simulink model "ntw4_3_2"  (R2018b)
settings: Solver=VariableStepAuto  StartTime=0.0  StopTime=10.0  RelTol=1e-3
settings Model: Creator=fyna  LastModifiedBy=fyna

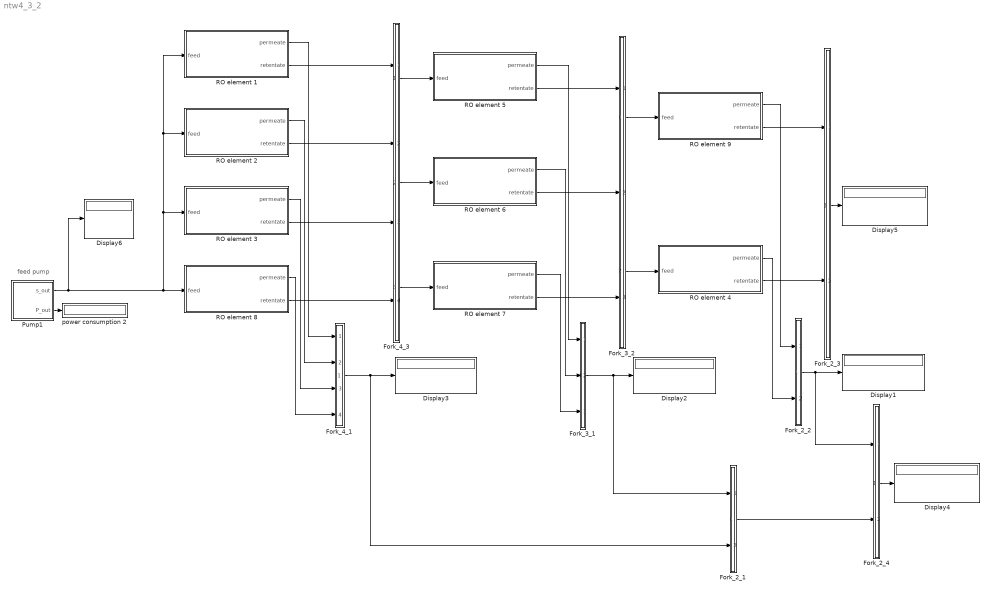
== system ntw4_3_2 ==
  note: feed pump
  Display{1..6} (6 alike) : Display
  Fork_2_1 : MATLAB Function  TreatAsAtomicUnit=on
  Fork_2_2 : MATLAB Function  TreatAsAtomicUnit=on
  Fork_2_3 : MATLAB Function  TreatAsAtomicUnit=on
  Fork_2_4 : MATLAB Function  TreatAsAtomicUnit=on
  Fork_3_1 : MATLAB Function  TreatAsAtomicUnit=on
  Fork_3_2 : MATLAB Function  TreatAsAtomicUnit=on
  Fork_4_1 : MATLAB Function  TreatAsAtomicUnit=on
  "Fork_4_3 " : MATLAB Function  TreatAsAtomicUnit=on
  Pump1 : Subsystem  mask(Hydraulic pump){q=6e3, p=15.5, c=0.0856, eta=0.8}
      mask prompts: q "volume flow rate [l/h]"; p "pressure [bar]"; c "concentration [mol/l]"; eta "efficiency"
      mask help: The hydraulic pump gerenates the hydrodynamic QPC state, through its embedded preferences. The power consumption is calculated as P = 3.6e-2*q*p/eta, [P] = kW.
      mask TypeOptions q: flow rate [l\h]/Value
      mask TypeOptions p: pressure [Pa]/Value
      mask TypeOptions c: concentration [mol//l]/Value
      mask TypeOptions eta: efficiency/Value
      mask Display: image("pumpSymbol2.png")
  RO element 1 : Subsystem  mask(8040 RO module){waterPerm=5, Value=0.995}
      mask prompts: waterPerm "water permeation coeff [lmh bar]]"; Value "salt rejection"
      mask help:
      | Reverse Osmosis module model. The permeate out-flow and feed out-flow are calculated from their respective in-flows and the membrane characteristics. A 28mil spacer is used in this module type.
      |
      | Input constants: membrane water permeability, salt rejection.
      mask TypeOptions waterPerm: waterPerm/Value
      mask TypeOptions Value: rejectionRate/Value
      mask Display: image('roSymbol.png');
  RO element 2 : Subsystem  mask(8040 RO module){waterPerm=5, Value=0.995}
      mask prompts: waterPerm "water permeation coeff [lmh bar]]"; Value "salt rejection"
      mask help:
      | Reverse Osmosis module model. The permeate out-flow and feed out-flow are calculated from their respective in-flows and the membrane characteristics. A 28mil spacer is used in this module type.
      |
      | Input constants: membrane water permeability, salt rejection.
      mask TypeOptions waterPerm: waterPerm/Value
      mask TypeOptions Value: rejectionRate/Value
      mask Display: image('roSymbol.png');
  RO element 3 : Subsystem  mask(8040 RO module){waterPerm=5, Value=0.995}
      mask prompts: waterPerm "water permeation coeff [lmh bar]]"; Value "salt rejection"
      mask help:
      | Reverse Osmosis module model. The permeate out-flow and feed out-flow are calculated from their respective in-flows and the membrane characteristics. A 28mil spacer is used in this module type.
      |
      | Input constants: membrane water permeability, salt rejection.
      mask TypeOptions waterPerm: waterPerm/Value
      mask TypeOptions Value: rejectionRate/Value
      mask Display: image('roSymbol.png');
  RO element 4 : Subsystem  mask(8040 RO module){waterPerm=5, Value=0.995}
      mask prompts: waterPerm "water permeation coeff [lmh bar]]"; Value "salt rejection"
      mask help:
      | Reverse Osmosis module model. The permeate out-flow and feed out-flow are calculated from their respective in-flows and the membrane characteristics. A 28mil spacer is used in this module type.
      |
      | Input constants: membrane water permeability, salt rejection.
      mask TypeOptions waterPerm: waterPerm/Value
      mask TypeOptions Value: rejectionRate/Value
      mask Display: image('roSymbol.png');
  RO element 5 : Subsystem  mask(8040 RO module){waterPerm=5, Value=0.995}
      mask prompts: waterPerm "water permeation coeff [lmh bar]]"; Value "salt rejection"
      mask help:
      | Reverse Osmosis module model. The permeate out-flow and feed out-flow are calculated from their respective in-flows and the membrane characteristics. A 28mil spacer is used in this module type.
      |
      | Input constants: membrane water permeability, salt rejection.
      mask TypeOptions waterPerm: waterPerm/Value
      mask TypeOptions Value: rejectionRate/Value
      mask Display: image('roSymbol.png');
  RO element 6 : Subsystem  mask(8040 RO module){waterPerm=5, Value=0.995}
      mask prompts: waterPerm "water permeation coeff [lmh bar]]"; Value "salt rejection"
      mask help:
      | Reverse Osmosis module model. The permeate out-flow and feed out-flow are calculated from their respective in-flows and the membrane characteristics. A 28mil spacer is used in this module type.
      |
      | Input constants: membrane water permeability, salt rejection.
      mask TypeOptions waterPerm: waterPerm/Value
      mask TypeOptions Value: rejectionRate/Value
      mask Display: image('roSymbol.png');
  RO element 7 : Subsystem  mask(8040 RO module){waterPerm=5, Value=0.995}
      mask prompts: waterPerm "water permeation coeff [lmh bar]]"; Value "salt rejection"
      mask help:
      | Reverse Osmosis module model. The permeate out-flow and feed out-flow are calculated from their respective in-flows and the membrane characteristics. A 28mil spacer is used in this module type.
      |
      | Input constants: membrane water permeability, salt rejection.
      mask TypeOptions waterPerm: waterPerm/Value
      mask TypeOptions Value: rejectionRate/Value
      mask Display: image('roSymbol.png');
  RO element 8 : Subsystem  mask(8040 RO module){waterPerm=5, Value=0.995}
      mask prompts: waterPerm "water permeation coeff [lmh bar]]"; Value "salt rejection"
      mask help:
      | Reverse Osmosis module model. The permeate out-flow and feed out-flow are calculated from their respective in-flows and the membrane characteristics. A 28mil spacer is used in this module type.
      |
      | Input constants: membrane water permeability, salt rejection.
      mask TypeOptions waterPerm: waterPerm/Value
      mask TypeOptions Value: rejectionRate/Value
      mask Display: image('roSymbol.png');
  RO element 9 : Subsystem  mask(8040 RO module){waterPerm=5, Value=0.995}
      mask prompts: waterPerm "water permeation coeff [lmh bar]]"; Value "salt rejection"
      mask help:
      | Reverse Osmosis module model. The permeate out-flow and feed out-flow are calculated from their respective in-flows and the membrane characteristics. A 28mil spacer is used in this module type.
      |
      | Input constants: membrane water permeability, salt rejection.
      mask TypeOptions waterPerm: waterPerm/Value
      mask TypeOptions Value: rejectionRate/Value
      mask Display: image('roSymbol.png');
  power consumption 2 : Display
  wires:
  RO element 8/2(retentate) -> "Fork_4_3 "/4(si_4)
  RO element 5/1(permeate) -> Fork_3_1/1(si_1)
  RO element 3/1(permeate) -> Fork_4_1/3(si_3)
  RO element 1/1(permeate) -> Fork_4_1/1(si_1)
  RO element 8/1(permeate) -> Fork_4_1/4(si_4)
  RO element 2/2(retentate) -> "Fork_4_3 "/2(si_2)
  Fork_4_1/1(so_1) -> Display3/1, Fork_2_1/2(si_2)
  Pump1/2(P_out) -> power consumption 2/1
  RO element 3/2(retentate) -> "Fork_4_3 "/3(si_3)
  Pump1/1(s_out) -> RO element 8/1(feed), RO element 3/1(feed), RO element 1/1(feed), RO element 2/1(feed), Display6/1
  RO element 1/2(retentate) -> "Fork_4_3 "/1(si_1)
  RO element 6/1(permeate) -> Fork_3_1/2(si_2)
  RO element 2/1(permeate) -> Fork_4_1/2(si_2)
  "Fork_4_3 "/1(so_1) -> RO element 5/1(feed)
  "Fork_4_3 "/2(so_2) -> RO element 6/1(feed)
  "Fork_4_3 "/3(so_3) -> RO element 7/1(feed)
  RO element 7/1(permeate) -> Fork_3_1/3(si_3)
  RO element 7/2(retentate) -> Fork_3_2/3(si_3)
  RO element 6/2(retentate) -> Fork_3_2/2(si_2)
  RO element 5/2(retentate) -> Fork_3_2/1(si_1)
  Fork_3_2/2(so_2) -> RO element 4/1(feed)
  Fork_3_2/1(so_1) -> RO element 9/1(feed)
  Fork_3_1/1(so_1) -> Display2/1, Fork_2_1/1(si_1)
  RO element 9/1(permeate) -> Fork_2_2/1(si_1)
  RO element 4/1(permeate) -> Fork_2_2/2(si_2)
  Fork_2_1/1(so_1) -> Fork_2_4/2(si_2)
  Fork_2_2/1(so_1) -> Display1/1, Fork_2_4/1(si_1)
  Fork_2_4/1(so_1) -> Display4/1
  RO element 9/2(retentate) -> Fork_2_3/1(si_1)
  RO element 4/2(retentate) -> Fork_2_3/2(si_2)
  Fork_2_3/1(so_1) -> Display5/1

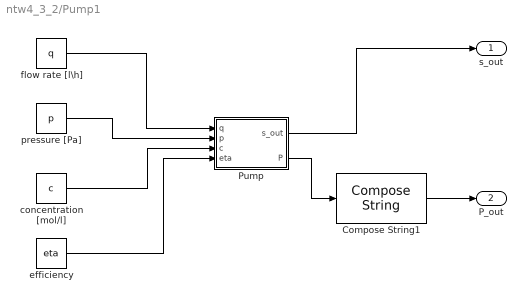
== system ntw4_3_2/Pump1 ==
  Compose String1 : ComposeString  Format='P = %.3f kW'
  Pump : MATLAB Function  TreatAsAtomicUnit=on
  concentration [mol/l] : Constant  Value=c
  efficiency : Constant  Value=eta
  flow rate [l\h] : Constant  Value=q
  pressure [Pa] : Constant  Value=p
  s_out : Outport
  P_out : Outport  Port=2
  wires:
  concentration [mol/l]/1 -> Pump/3(c)
  flow rate [l\h]/1 -> Pump/1(q)
  Pump/1(s_out) -> s_out/1
  pressure [Pa]/1 -> Pump/2(p)
  efficiency/1 -> Pump/4(eta)
  Compose String1/1 -> P_out/1
  Pump/2(P) -> Compose String1/1

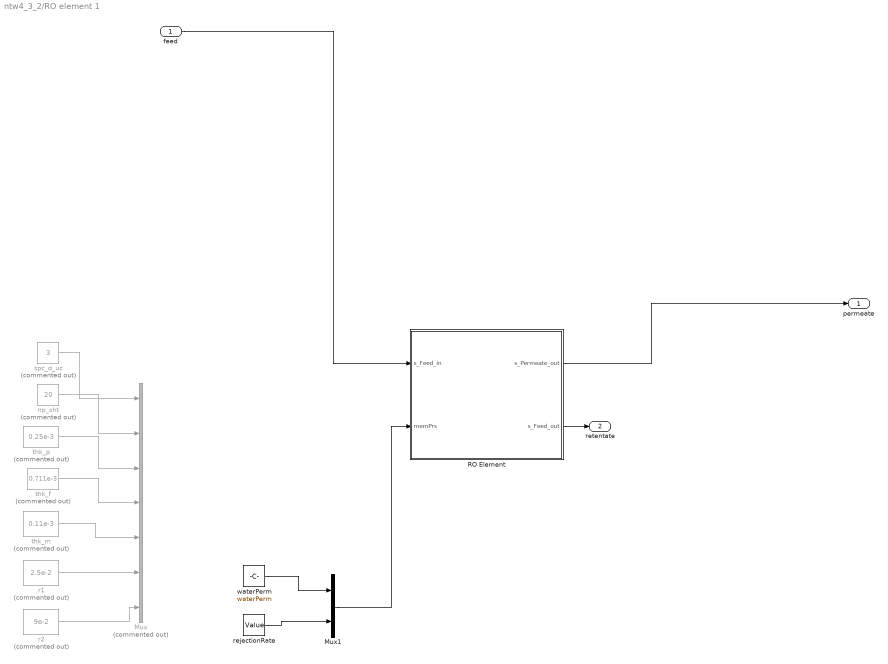
== system ntw4_3_2/RO element 1 ==
  feed : Inport
  Mux : Mux  Commented=on  Inputs=7
  Mux1 : Mux  Inputs=2
  RO Element : MATLAB Function  TreatAsAtomicUnit=on
  np_sht : Constant  Commented=on  Value=20
  r1 : Constant  Commented=on  Value=2.5e-2
  r2 : Constant  Commented=on  Value=9e-2
  rejectionRate : Constant  Value=Value
  spc_d_uc : Constant  Commented=on  Value=3
  thk_f : Constant  Commented=on  Value=0.711e-3
  thk_m : Constant  Commented=on  Value=0.11e-3
  thk_p : Constant  Commented=on  Value=0.25e-3
  waterPerm : Constant  Value=waterPerm
  permeate : Outport
  retentate : Outport  Port=2
  wires:
  spc_d_uc/1 -> Mux/1
  feed/1 -> RO Element/1(s_Feed_in)
  waterPerm/1 -> Mux1/1
  r1/1 -> Mux/6
  thk_m/1 -> Mux/5
  Mux1/1 -> RO Element/2(memPrs)
  r2/1 -> Mux/7
  RO Element/2(s_Feed_out) -> retentate/1
  rejectionRate/1 -> Mux1/2
  RO Element/1(s_Permeate_out) -> permeate/1
  thk_p/1 -> Mux/3
  thk_f/1 -> Mux/4
  np_sht/1 -> Mux/2

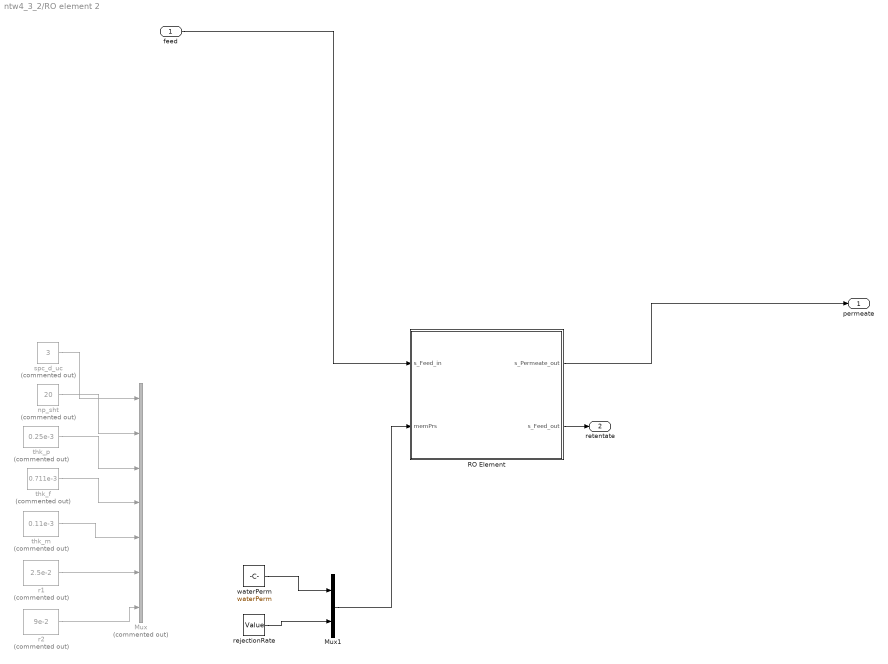
== system ntw4_3_2/RO element 2 ==
  feed : Inport
  Mux : Mux  Commented=on  Inputs=7
  Mux1 : Mux  Inputs=2
  RO Element : MATLAB Function  TreatAsAtomicUnit=on
  np_sht : Constant  Commented=on  Value=20
  r1 : Constant  Commented=on  Value=2.5e-2
  r2 : Constant  Commented=on  Value=9e-2
  rejectionRate : Constant  Value=Value
  spc_d_uc : Constant  Commented=on  Value=3
  thk_f : Constant  Commented=on  Value=0.711e-3
  thk_m : Constant  Commented=on  Value=0.11e-3
  thk_p : Constant  Commented=on  Value=0.25e-3
  waterPerm : Constant  Value=waterPerm
  permeate : Outport
  retentate : Outport  Port=2
  wires:
  spc_d_uc/1 -> Mux/1
  feed/1 -> RO Element/1(s_Feed_in)
  waterPerm/1 -> Mux1/1
  r1/1 -> Mux/6
  thk_m/1 -> Mux/5
  Mux1/1 -> RO Element/2(memPrs)
  r2/1 -> Mux/7
  RO Element/2(s_Feed_out) -> retentate/1
  rejectionRate/1 -> Mux1/2
  RO Element/1(s_Permeate_out) -> permeate/1
  thk_p/1 -> Mux/3
  thk_f/1 -> Mux/4
  np_sht/1 -> Mux/2

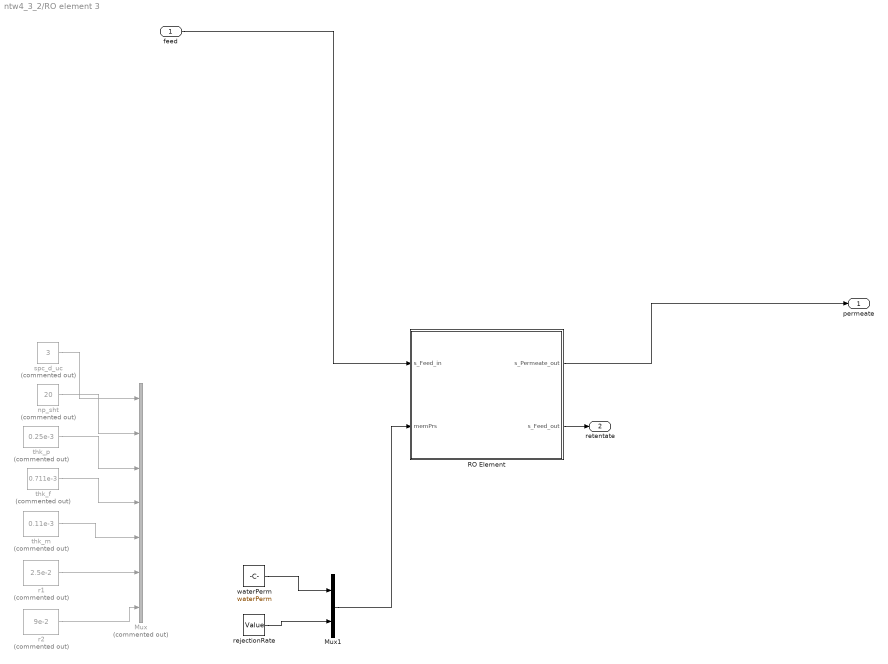
== system ntw4_3_2/RO element 3 ==
  feed : Inport
  Mux : Mux  Commented=on  Inputs=7
  Mux1 : Mux  Inputs=2
  RO Element : MATLAB Function  TreatAsAtomicUnit=on
  np_sht : Constant  Commented=on  Value=20
  r1 : Constant  Commented=on  Value=2.5e-2
  r2 : Constant  Commented=on  Value=9e-2
  rejectionRate : Constant  Value=Value
  spc_d_uc : Constant  Commented=on  Value=3
  thk_f : Constant  Commented=on  Value=0.711e-3
  thk_m : Constant  Commented=on  Value=0.11e-3
  thk_p : Constant  Commented=on  Value=0.25e-3
  waterPerm : Constant  Value=waterPerm
  permeate : Outport
  retentate : Outport  Port=2
  wires:
  spc_d_uc/1 -> Mux/1
  feed/1 -> RO Element/1(s_Feed_in)
  waterPerm/1 -> Mux1/1
  r1/1 -> Mux/6
  thk_m/1 -> Mux/5
  Mux1/1 -> RO Element/2(memPrs)
  r2/1 -> Mux/7
  RO Element/2(s_Feed_out) -> retentate/1
  rejectionRate/1 -> Mux1/2
  RO Element/1(s_Permeate_out) -> permeate/1
  thk_p/1 -> Mux/3
  thk_f/1 -> Mux/4
  np_sht/1 -> Mux/2

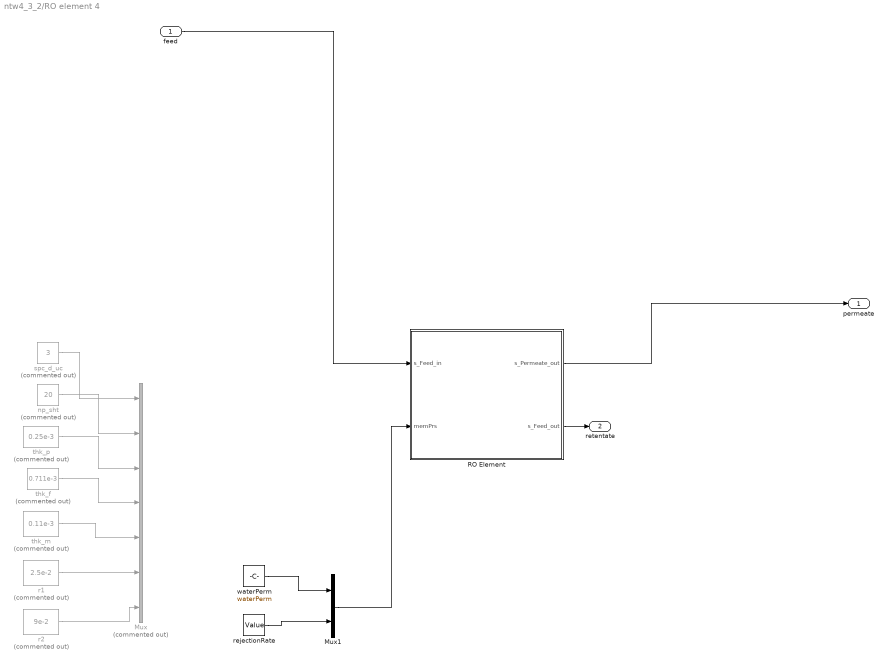
== system ntw4_3_2/RO element 4 ==
  feed : Inport
  Mux : Mux  Commented=on  Inputs=7
  Mux1 : Mux  Inputs=2
  RO Element : MATLAB Function  TreatAsAtomicUnit=on
  np_sht : Constant  Commented=on  Value=20
  r1 : Constant  Commented=on  Value=2.5e-2
  r2 : Constant  Commented=on  Value=9e-2
  rejectionRate : Constant  Value=Value
  spc_d_uc : Constant  Commented=on  Value=3
  thk_f : Constant  Commented=on  Value=0.711e-3
  thk_m : Constant  Commented=on  Value=0.11e-3
  thk_p : Constant  Commented=on  Value=0.25e-3
  waterPerm : Constant  Value=waterPerm
  permeate : Outport
  retentate : Outport  Port=2
  wires:
  spc_d_uc/1 -> Mux/1
  feed/1 -> RO Element/1(s_Feed_in)
  waterPerm/1 -> Mux1/1
  r1/1 -> Mux/6
  thk_m/1 -> Mux/5
  Mux1/1 -> RO Element/2(memPrs)
  r2/1 -> Mux/7
  RO Element/2(s_Feed_out) -> retentate/1
  rejectionRate/1 -> Mux1/2
  RO Element/1(s_Permeate_out) -> permeate/1
  thk_p/1 -> Mux/3
  thk_f/1 -> Mux/4
  np_sht/1 -> Mux/2

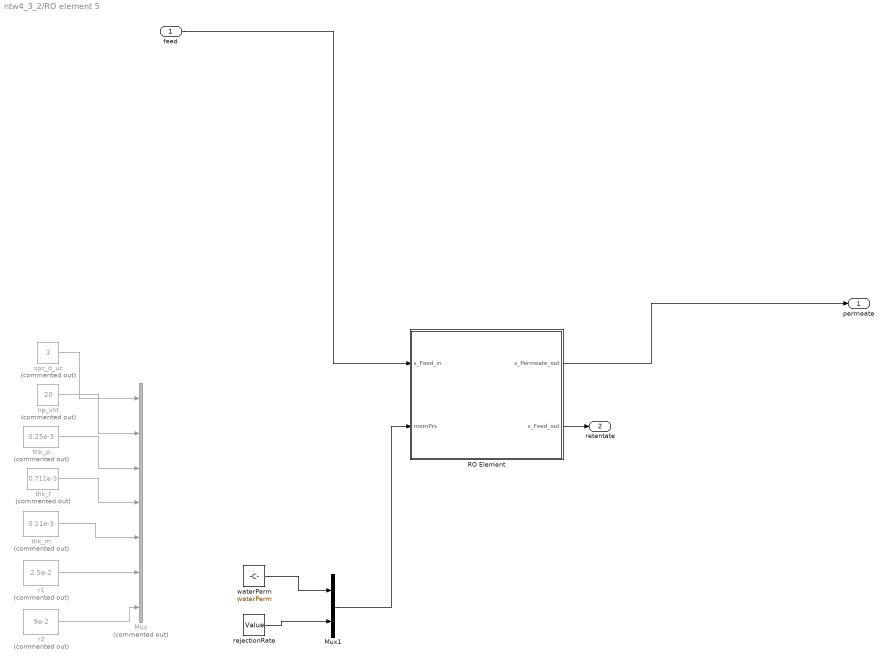
== system ntw4_3_2/RO element 5 ==
  feed : Inport
  Mux : Mux  Commented=on  Inputs=7
  Mux1 : Mux  Inputs=2
  RO Element : MATLAB Function  TreatAsAtomicUnit=on
  np_sht : Constant  Commented=on  Value=20
  r1 : Constant  Commented=on  Value=2.5e-2
  r2 : Constant  Commented=on  Value=9e-2
  rejectionRate : Constant  Value=Value
  spc_d_uc : Constant  Commented=on  Value=3
  thk_f : Constant  Commented=on  Value=0.711e-3
  thk_m : Constant  Commented=on  Value=0.11e-3
  thk_p : Constant  Commented=on  Value=0.25e-3
  waterPerm : Constant  Value=waterPerm
  permeate : Outport
  retentate : Outport  Port=2
  wires:
  spc_d_uc/1 -> Mux/1
  feed/1 -> RO Element/1(s_Feed_in)
  waterPerm/1 -> Mux1/1
  r1/1 -> Mux/6
  thk_m/1 -> Mux/5
  Mux1/1 -> RO Element/2(memPrs)
  r2/1 -> Mux/7
  RO Element/2(s_Feed_out) -> retentate/1
  rejectionRate/1 -> Mux1/2
  RO Element/1(s_Permeate_out) -> permeate/1
  thk_p/1 -> Mux/3
  thk_f/1 -> Mux/4
  np_sht/1 -> Mux/2

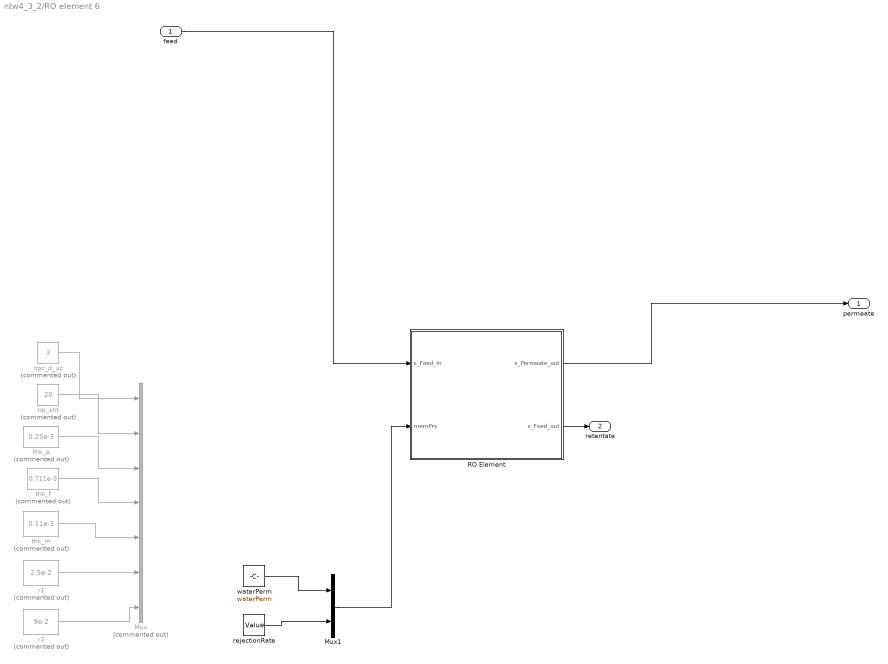
== system ntw4_3_2/RO element 6 ==
  feed : Inport
  Mux : Mux  Commented=on  Inputs=7
  Mux1 : Mux  Inputs=2
  RO Element : MATLAB Function  TreatAsAtomicUnit=on
  np_sht : Constant  Commented=on  Value=20
  r1 : Constant  Commented=on  Value=2.5e-2
  r2 : Constant  Commented=on  Value=9e-2
  rejectionRate : Constant  Value=Value
  spc_d_uc : Constant  Commented=on  Value=3
  thk_f : Constant  Commented=on  Value=0.711e-3
  thk_m : Constant  Commented=on  Value=0.11e-3
  thk_p : Constant  Commented=on  Value=0.25e-3
  waterPerm : Constant  Value=waterPerm
  permeate : Outport
  retentate : Outport  Port=2
  wires:
  spc_d_uc/1 -> Mux/1
  feed/1 -> RO Element/1(s_Feed_in)
  waterPerm/1 -> Mux1/1
  r1/1 -> Mux/6
  thk_m/1 -> Mux/5
  Mux1/1 -> RO Element/2(memPrs)
  r2/1 -> Mux/7
  RO Element/2(s_Feed_out) -> retentate/1
  rejectionRate/1 -> Mux1/2
  RO Element/1(s_Permeate_out) -> permeate/1
  thk_p/1 -> Mux/3
  thk_f/1 -> Mux/4
  np_sht/1 -> Mux/2

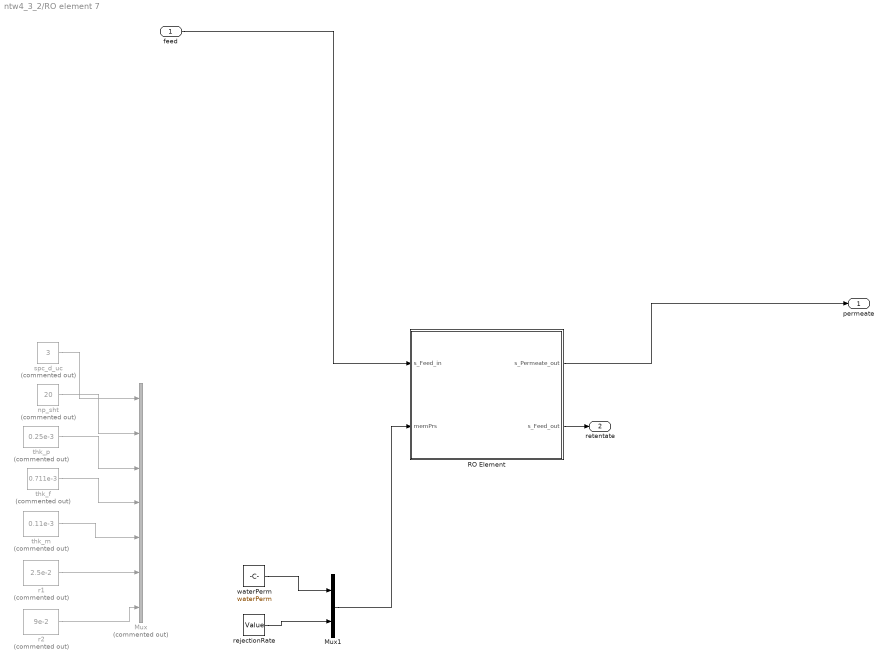
== system ntw4_3_2/RO element 7 ==
  feed : Inport
  Mux : Mux  Commented=on  Inputs=7
  Mux1 : Mux  Inputs=2
  RO Element : MATLAB Function  TreatAsAtomicUnit=on
  np_sht : Constant  Commented=on  Value=20
  r1 : Constant  Commented=on  Value=2.5e-2
  r2 : Constant  Commented=on  Value=9e-2
  rejectionRate : Constant  Value=Value
  spc_d_uc : Constant  Commented=on  Value=3
  thk_f : Constant  Commented=on  Value=0.711e-3
  thk_m : Constant  Commented=on  Value=0.11e-3
  thk_p : Constant  Commented=on  Value=0.25e-3
  waterPerm : Constant  Value=waterPerm
  permeate : Outport
  retentate : Outport  Port=2
  wires:
  spc_d_uc/1 -> Mux/1
  feed/1 -> RO Element/1(s_Feed_in)
  waterPerm/1 -> Mux1/1
  r1/1 -> Mux/6
  thk_m/1 -> Mux/5
  Mux1/1 -> RO Element/2(memPrs)
  r2/1 -> Mux/7
  RO Element/2(s_Feed_out) -> retentate/1
  rejectionRate/1 -> Mux1/2
  RO Element/1(s_Permeate_out) -> permeate/1
  thk_p/1 -> Mux/3
  thk_f/1 -> Mux/4
  np_sht/1 -> Mux/2

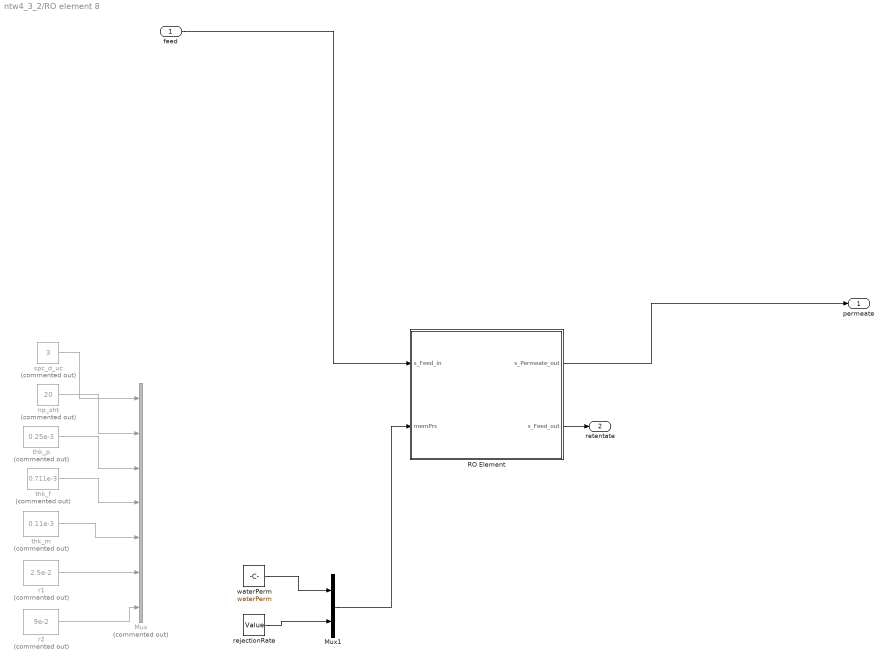
== system ntw4_3_2/RO element 8 ==
  feed : Inport
  Mux : Mux  Commented=on  Inputs=7
  Mux1 : Mux  Inputs=2
  RO Element : MATLAB Function  TreatAsAtomicUnit=on
  np_sht : Constant  Commented=on  Value=20
  r1 : Constant  Commented=on  Value=2.5e-2
  r2 : Constant  Commented=on  Value=9e-2
  rejectionRate : Constant  Value=Value
  spc_d_uc : Constant  Commented=on  Value=3
  thk_f : Constant  Commented=on  Value=0.711e-3
  thk_m : Constant  Commented=on  Value=0.11e-3
  thk_p : Constant  Commented=on  Value=0.25e-3
  waterPerm : Constant  Value=waterPerm
  permeate : Outport
  retentate : Outport  Port=2
  wires:
  spc_d_uc/1 -> Mux/1
  feed/1 -> RO Element/1(s_Feed_in)
  waterPerm/1 -> Mux1/1
  r1/1 -> Mux/6
  thk_m/1 -> Mux/5
  Mux1/1 -> RO Element/2(memPrs)
  r2/1 -> Mux/7
  RO Element/2(s_Feed_out) -> retentate/1
  rejectionRate/1 -> Mux1/2
  RO Element/1(s_Permeate_out) -> permeate/1
  thk_p/1 -> Mux/3
  thk_f/1 -> Mux/4
  np_sht/1 -> Mux/2

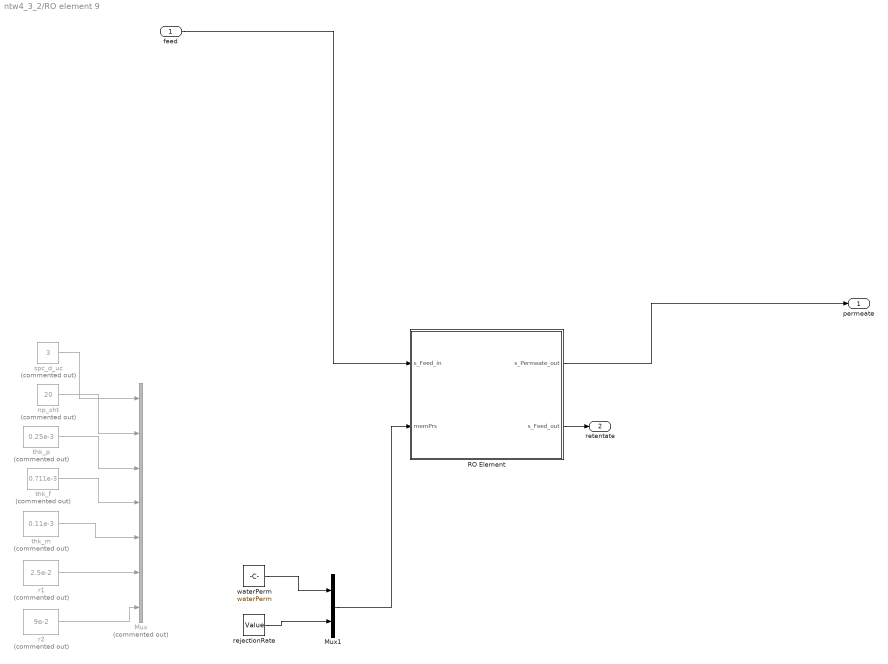
== system ntw4_3_2/RO element 9 ==
  feed : Inport
  Mux : Mux  Commented=on  Inputs=7
  Mux1 : Mux  Inputs=2
  RO Element : MATLAB Function  TreatAsAtomicUnit=on
  np_sht : Constant  Commented=on  Value=20
  r1 : Constant  Commented=on  Value=2.5e-2
  r2 : Constant  Commented=on  Value=9e-2
  rejectionRate : Constant  Value=Value
  spc_d_uc : Constant  Commented=on  Value=3
  thk_f : Constant  Commented=on  Value=0.711e-3
  thk_m : Constant  Commented=on  Value=0.11e-3
  thk_p : Constant  Commented=on  Value=0.25e-3
  waterPerm : Constant  Value=waterPerm
  permeate : Outport
  retentate : Outport  Port=2
  wires:
  spc_d_uc/1 -> Mux/1
  feed/1 -> RO Element/1(s_Feed_in)
  waterPerm/1 -> Mux1/1
  r1/1 -> Mux/6
  thk_m/1 -> Mux/5
  Mux1/1 -> RO Element/2(memPrs)
  r2/1 -> Mux/7
  RO Element/2(s_Feed_out) -> retentate/1
  rejectionRate/1 -> Mux1/2
  RO Element/1(s_Permeate_out) -> permeate/1
  thk_p/1 -> Mux/3
  thk_f/1 -> Mux/4
  np_sht/1 -> Mux/2

== matlab function ntw4_3_2/RO element 1/RO Element ==
  data: s_Feed_in input; s_Permeate_out output; s_Feed_out output; memPrs input
function [s_Permeate_out, s_Feed_out] = fcn(s_Feed_in, memPrs)

% moduleParas = [d_uc, no_sht, thk_d, thk_f, thk_m, r1, r2]

% ---------------------------------fixing flow rate:
nbSheets = 20;
l_s     = 1.1;
l_l     = 0.93;

q_in    = s_Feed_in(1)/3.6*1e-6;        %m^3/s
U       = q_in/(l_s*0.711e-3*nbSheets);

dh      = 1.0673e-3;        % m
re      = U*dh*1e6;
sh      = 4.43655*re^0.48267;
D       = 1.45e-9;          % m^2/s
k_m     = sh*D/dh;        

A_m     = memPrs(1)/3.6*1e-11;  % m/s/pa
zeta    = 8.05e4;               % pa m^3/kg
molarMassNaCl   = 58.44276;     % g/mol
c_f     = s_Feed_in(3)*molarMassNaCl;       %g/l
%c_p     = s_Permeate_in(3)*molarMassNaCl;   %g/l
d_p     = s_Feed_in(2)*1e5;  % pa

a   = 0.0;
b   = 1e-4;
%fprintf('A_m = %e, dp = %e, u = %e, re = %e, k_m = %e, sh = %e\n', A_m, d_p, U, re, k_m, sh);
while abs(a-b) > 1e-10
    x   = 0.5*(a+b);
    fa  = a - A_m*(  d_p - zeta*( c_f*exp(a/k_m) )  );
    fx  = x - A_m*(  d_p - zeta*( c_f*exp(x/k_m) )  );
    %fprintf('a = %e, b = %e, x = %e, abs(a-b) = %e\n',a,b,x, abs(a-b));

    if fa*fx>0
        a   = x;
    else
        b   = x;
    end
end
jw_uc   = 0.5*(a+b);

n_s = round(l_s/(2.822e-3));
n_l = round(l_l/(2.822e-3));
area_uc = 16e-6;                %m^2
area_mod = area_uc*n_s*n_l*nbSheets;

q_mem = area_mod*jw_uc;         % m^3/s


% ---------------------------------fixing solute flux:
R_m   = memPrs(2);
q_s_m = q_mem*c_f*(1.0-R_m);    % kg/m^3, solute mass flow rate through membrane
q_s_r = (q_in*c_f - q_s_m);     % kg/m^3, solute mass flow rate retained in feed channel

% ---------------------------------fixing pressure drop:
f       = 22.91*re^-0.606;
dP      = f*U^2*1e3*l_l/(2.0*dh)*1e-5;  % bar
fprintf('f = %e\n',area_mod);

q_feed_out = (q_in-q_mem)*3.6e6 ;
p_feed_out = s_Feed_in(2) - dP;
c_feed_out = q_s_r/(q_feed_out/3.6e6)/molarMassNaCl;

q_perm_out = q_mem*3.6e6;      %l/h
p_perm_out = 0;
c_perm_out = q_s_m/q_mem/molarMassNaCl;

s_Feed_out      = [q_feed_out, p_feed_out, c_feed_out];
s_Permeate_out  = [q_perm_out, p_perm_out, c_perm_out];

== matlab function ntw4_3_2/RO element 2/RO Element ==
  data: s_Feed_in input; s_Permeate_out output; s_Feed_out output; memPrs input
function [s_Permeate_out, s_Feed_out] = fcn(s_Feed_in, memPrs)

% moduleParas = [d_uc, no_sht, thk_d, thk_f, thk_m, r1, r2]

% ---------------------------------fixing flow rate:
nbSheets = 20;
l_s     = 1.1;
l_l     = 0.93;

q_in    = s_Feed_in(1)/3.6*1e-6;        %m^3/s
U       = q_in/(l_s*0.711e-3*nbSheets);

dh      = 1.0673e-3;        % m
re      = U*dh*1e6;
sh      = 4.43655*re^0.48267;
D       = 1.45e-9;          % m^2/s
k_m     = sh*D/dh;        

A_m     = memPrs(1)/3.6*1e-11;  % m/s/pa
zeta    = 8.05e4;               % pa m^3/kg
molarMassNaCl   = 58.44276;     % g/mol
c_f     = s_Feed_in(3)*molarMassNaCl;       %g/l
%c_p     = s_Permeate_in(3)*molarMassNaCl;   %g/l
d_p     = s_Feed_in(2)*1e5;  % pa

a   = 0.0;
b   = 1e-4;
%fprintf('A_m = %e, dp = %e, u = %e, re = %e, k_m = %e, sh = %e\n', A_m, d_p, U, re, k_m, sh);
while abs(a-b) > 1e-10
    x   = 0.5*(a+b);
    fa  = a - A_m*(  d_p - zeta*( c_f*exp(a/k_m) )  );
    fx  = x - A_m*(  d_p - zeta*( c_f*exp(x/k_m) )  );
    %fprintf('a = %e, b = %e, x = %e, abs(a-b) = %e\n',a,b,x, abs(a-b));

    if fa*fx>0
        a   = x;
    else
        b   = x;
    end
end
jw_uc   = 0.5*(a+b);

n_s = round(l_s/(2.822e-3));
n_l = round(l_l/(2.822e-3));
area_uc = 16e-6;                %m^2
area_mod = area_uc*n_s*n_l*nbSheets;

q_mem = area_mod*jw_uc;         % m^3/s


% ---------------------------------fixing solute flux:
R_m   = memPrs(2);
q_s_m = q_mem*c_f*(1.0-R_m);    % kg/m^3, solute mass flow rate through membrane
q_s_r = (q_in*c_f - q_s_m);     % kg/m^3, solute mass flow rate retained in feed channel

% ---------------------------------fixing pressure drop:
f       = 22.91*re^-0.606;
dP      = f*U^2*1e3*l_l/(2.0*dh)*1e-5;  % bar
fprintf('f = %e\n',area_mod);

q_feed_out = (q_in-q_mem)*3.6e6 ;
p_feed_out = s_Feed_in(2) - dP;
c_feed_out = q_s_r/(q_feed_out/3.6e6)/molarMassNaCl;

q_perm_out = q_mem*3.6e6;      %l/h
p_perm_out = 0;
c_perm_out = q_s_m/q_mem/molarMassNaCl;

s_Feed_out      = [q_feed_out, p_feed_out, c_feed_out];
s_Permeate_out  = [q_perm_out, p_perm_out, c_perm_out];

== matlab function ntw4_3_2/Pump1/Pump ==
  data: q input; s_out output; p input; c input; eta input; P output
function [s_out,P ] = fcn(q,p,c,eta)

P = q*p/eta/3.6e4;     % power consumption in kW
s_out = [q,p,c];

== matlab function ntw4_3_2/RO element 3/RO Element ==
  data: s_Feed_in input; s_Permeate_out output; s_Feed_out output; memPrs input
function [s_Permeate_out, s_Feed_out] = fcn(s_Feed_in, memPrs)

% moduleParas = [d_uc, no_sht, thk_d, thk_f, thk_m, r1, r2]

% ---------------------------------fixing flow rate:
nbSheets = 20;
l_s     = 1.1;
l_l     = 0.93;

q_in    = s_Feed_in(1)/3.6*1e-6;        %m^3/s
U       = q_in/(l_s*0.711e-3*nbSheets);

dh      = 1.0673e-3;        % m
re      = U*dh*1e6;
sh      = 4.43655*re^0.48267;
D       = 1.45e-9;          % m^2/s
k_m     = sh*D/dh;        

A_m     = memPrs(1)/3.6*1e-11;  % m/s/pa
zeta    = 8.05e4;               % pa m^3/kg
molarMassNaCl   = 58.44276;     % g/mol
c_f     = s_Feed_in(3)*molarMassNaCl;       %g/l
%c_p     = s_Permeate_in(3)*molarMassNaCl;   %g/l
d_p     = s_Feed_in(2)*1e5;  % pa

a   = 0.0;
b   = 1e-4;
%fprintf('A_m = %e, dp = %e, u = %e, re = %e, k_m = %e, sh = %e\n', A_m, d_p, U, re, k_m, sh);
while abs(a-b) > 1e-10
    x   = 0.5*(a+b);
    fa  = a - A_m*(  d_p - zeta*( c_f*exp(a/k_m) )  );
    fx  = x - A_m*(  d_p - zeta*( c_f*exp(x/k_m) )  );
    %fprintf('a = %e, b = %e, x = %e, abs(a-b) = %e\n',a,b,x, abs(a-b));

    if fa*fx>0
        a   = x;
    else
        b   = x;
    end
end
jw_uc   = 0.5*(a+b);

n_s = round(l_s/(2.822e-3));
n_l = round(l_l/(2.822e-3));
area_uc = 16e-6;                %m^2
area_mod = area_uc*n_s*n_l*nbSheets;

q_mem = area_mod*jw_uc;         % m^3/s


% ---------------------------------fixing solute flux:
R_m   = memPrs(2);
q_s_m = q_mem*c_f*(1.0-R_m);    % kg/m^3, solute mass flow rate through membrane
q_s_r = (q_in*c_f - q_s_m);     % kg/m^3, solute mass flow rate retained in feed channel

% ---------------------------------fixing pressure drop:
f       = 22.91*re^-0.606;
dP      = f*U^2*1e3*l_l/(2.0*dh)*1e-5;  % bar
fprintf('f = %e\n',area_mod);

q_feed_out = (q_in-q_mem)*3.6e6 ;
p_feed_out = s_Feed_in(2) - dP;
c_feed_out = q_s_r/(q_feed_out/3.6e6)/molarMassNaCl;

q_perm_out = q_mem*3.6e6;      %l/h
p_perm_out = 0;
c_perm_out = q_s_m/q_mem/molarMassNaCl;

s_Feed_out      = [q_feed_out, p_feed_out, c_feed_out];
s_Permeate_out  = [q_perm_out, p_perm_out, c_perm_out];

== matlab function ntw4_3_2/RO element 9/RO Element ==
  data: s_Feed_in input; s_Permeate_out output; s_Feed_out output; memPrs input
function [s_Permeate_out, s_Feed_out] = fcn(s_Feed_in, memPrs)

% moduleParas = [d_uc, no_sht, thk_d, thk_f, thk_m, r1, r2]

% ---------------------------------fixing flow rate:
nbSheets = 20;
l_s     = 1.1;
l_l     = 0.93;

q_in    = s_Feed_in(1)/3.6*1e-6;        %m^3/s
U       = q_in/(l_s*0.711e-3*nbSheets);

dh      = 1.0673e-3;        % m
re      = U*dh*1e6;
sh      = 4.43655*re^0.48267;
D       = 1.45e-9;          % m^2/s
k_m     = sh*D/dh;        

A_m     = memPrs(1)/3.6*1e-11;  % m/s/pa
zeta    = 8.05e4;               % pa m^3/kg
molarMassNaCl   = 58.44276;     % g/mol
c_f     = s_Feed_in(3)*molarMassNaCl;       %g/l
%c_p     = s_Permeate_in(3)*molarMassNaCl;   %g/l
d_p     = s_Feed_in(2)*1e5;  % pa

a   = 0.0;
b   = 1e-4;
%fprintf('A_m = %e, dp = %e, u = %e, re = %e, k_m = %e, sh = %e\n', A_m, d_p, U, re, k_m, sh);
while abs(a-b) > 1e-10
    x   = 0.5*(a+b);
    fa  = a - A_m*(  d_p - zeta*( c_f*exp(a/k_m) )  );
    fx  = x - A_m*(  d_p - zeta*( c_f*exp(x/k_m) )  );
    %fprintf('a = %e, b = %e, x = %e, abs(a-b) = %e\n',a,b,x, abs(a-b));

    if fa*fx>0
        a   = x;
    else
        b   = x;
    end
end
jw_uc   = 0.5*(a+b);

n_s = round(l_s/(2.822e-3));
n_l = round(l_l/(2.822e-3));
area_uc = 16e-6;                %m^2
area_mod = area_uc*n_s*n_l*nbSheets;

q_mem = area_mod*jw_uc;         % m^3/s


% ---------------------------------fixing solute flux:
R_m   = memPrs(2);
q_s_m = q_mem*c_f*(1.0-R_m);    % kg/m^3, solute mass flow rate through membrane
q_s_r = (q_in*c_f - q_s_m);     % kg/m^3, solute mass flow rate retained in feed channel

% ---------------------------------fixing pressure drop:
f       = 22.91*re^-0.606;
dP      = f*U^2*1e3*l_l/(2.0*dh)*1e-5;  % bar
fprintf('f = %e\n',area_mod);

q_feed_out = (q_in-q_mem)*3.6e6 ;
p_feed_out = s_Feed_in(2) - dP;
c_feed_out = q_s_r/(q_feed_out/3.6e6)/molarMassNaCl;

q_perm_out = q_mem*3.6e6;      %l/h
p_perm_out = 0;
c_perm_out = q_s_m/q_mem/molarMassNaCl;

s_Feed_out      = [q_feed_out, p_feed_out, c_feed_out];
s_Permeate_out  = [q_perm_out, p_perm_out, c_perm_out];

== matlab function ntw4_3_2/RO element 8/RO Element ==
  data: s_Feed_in input; s_Permeate_out output; s_Feed_out output; memPrs input
function [s_Permeate_out, s_Feed_out] = fcn(s_Feed_in, memPrs)

% moduleParas = [d_uc, no_sht, thk_d, thk_f, thk_m, r1, r2]

% ---------------------------------fixing flow rate:
nbSheets = 20;
l_s     = 1.1;
l_l     = 0.93;

q_in    = s_Feed_in(1)/3.6*1e-6;        %m^3/s
U       = q_in/(l_s*0.711e-3*nbSheets);

dh      = 1.0673e-3;        % m
re      = U*dh*1e6;
sh      = 4.43655*re^0.48267;
D       = 1.45e-9;          % m^2/s
k_m     = sh*D/dh;        

A_m     = memPrs(1)/3.6*1e-11;  % m/s/pa
zeta    = 8.05e4;               % pa m^3/kg
molarMassNaCl   = 58.44276;     % g/mol
c_f     = s_Feed_in(3)*molarMassNaCl;       %g/l
%c_p     = s_Permeate_in(3)*molarMassNaCl;   %g/l
d_p     = s_Feed_in(2)*1e5;  % pa

a   = 0.0;
b   = 1e-4;
%fprintf('A_m = %e, dp = %e, u = %e, re = %e, k_m = %e, sh = %e\n', A_m, d_p, U, re, k_m, sh);
while abs(a-b) > 1e-10
    x   = 0.5*(a+b);
    fa  = a - A_m*(  d_p - zeta*( c_f*exp(a/k_m) )  );
    fx  = x - A_m*(  d_p - zeta*( c_f*exp(x/k_m) )  );
    %fprintf('a = %e, b = %e, x = %e, abs(a-b) = %e\n',a,b,x, abs(a-b));

    if fa*fx>0
        a   = x;
    else
        b   = x;
    end
end
jw_uc   = 0.5*(a+b);

n_s = round(l_s/(2.822e-3));
n_l = round(l_l/(2.822e-3));
area_uc = 16e-6;                %m^2
area_mod = area_uc*n_s*n_l*nbSheets;

q_mem = area_mod*jw_uc;         % m^3/s


% ---------------------------------fixing solute flux:
R_m   = memPrs(2);
q_s_m = q_mem*c_f*(1.0-R_m);    % kg/m^3, solute mass flow rate through membrane
q_s_r = (q_in*c_f - q_s_m);     % kg/m^3, solute mass flow rate retained in feed channel

% ---------------------------------fixing pressure drop:
f       = 22.91*re^-0.606;
dP      = f*U^2*1e3*l_l/(2.0*dh)*1e-5;  % bar
fprintf('f = %e\n',area_mod);

q_feed_out = (q_in-q_mem)*3.6e6 ;
p_feed_out = s_Feed_in(2) - dP;
c_feed_out = q_s_r/(q_feed_out/3.6e6)/molarMassNaCl;

q_perm_out = q_mem*3.6e6;      %l/h
p_perm_out = 0;
c_perm_out = q_s_m/q_mem/molarMassNaCl;

s_Feed_out      = [q_feed_out, p_feed_out, c_feed_out];
s_Permeate_out  = [q_perm_out, p_perm_out, c_perm_out];

== matlab function ntw4_3_2/RO element 4/RO Element ==
  data: s_Feed_in input; s_Permeate_out output; s_Feed_out output; memPrs input
function [s_Permeate_out, s_Feed_out] = fcn(s_Feed_in, memPrs)

% moduleParas = [d_uc, no_sht, thk_d, thk_f, thk_m, r1, r2]

% ---------------------------------fixing flow rate:
nbSheets = 20;
l_s     = 1.1;
l_l     = 0.93;

q_in    = s_Feed_in(1)/3.6*1e-6;        %m^3/s
U       = q_in/(l_s*0.711e-3*nbSheets);

dh      = 1.0673e-3;        % m
re      = U*dh*1e6;
sh      = 4.43655*re^0.48267;
D       = 1.45e-9;          % m^2/s
k_m     = sh*D/dh;        

A_m     = memPrs(1)/3.6*1e-11;  % m/s/pa
zeta    = 8.05e4;               % pa m^3/kg
molarMassNaCl   = 58.44276;     % g/mol
c_f     = s_Feed_in(3)*molarMassNaCl;       %g/l
%c_p     = s_Permeate_in(3)*molarMassNaCl;   %g/l
d_p     = s_Feed_in(2)*1e5;  % pa

a   = 0.0;
b   = 1e-4;
%fprintf('A_m = %e, dp = %e, u = %e, re = %e, k_m = %e, sh = %e\n', A_m, d_p, U, re, k_m, sh);
while abs(a-b) > 1e-10
    x   = 0.5*(a+b);
    fa  = a - A_m*(  d_p - zeta*( c_f*exp(a/k_m) )  );
    fx  = x - A_m*(  d_p - zeta*( c_f*exp(x/k_m) )  );
    %fprintf('a = %e, b = %e, x = %e, abs(a-b) = %e\n',a,b,x, abs(a-b));

    if fa*fx>0
        a   = x;
    else
        b   = x;
    end
end
jw_uc   = 0.5*(a+b);

n_s = round(l_s/(2.822e-3));
n_l = round(l_l/(2.822e-3));
area_uc = 16e-6;                %m^2
area_mod = area_uc*n_s*n_l*nbSheets;

q_mem = area_mod*jw_uc;         % m^3/s


% ---------------------------------fixing solute flux:
R_m   = memPrs(2);
q_s_m = q_mem*c_f*(1.0-R_m);    % kg/m^3, solute mass flow rate through membrane
q_s_r = (q_in*c_f - q_s_m);     % kg/m^3, solute mass flow rate retained in feed channel

% ---------------------------------fixing pressure drop:
f       = 22.91*re^-0.606;
dP      = f*U^2*1e3*l_l/(2.0*dh)*1e-5;  % bar
fprintf('f = %e\n',area_mod);

q_feed_out = (q_in-q_mem)*3.6e6 ;
p_feed_out = s_Feed_in(2) - dP;
c_feed_out = q_s_r/(q_feed_out/3.6e6)/molarMassNaCl;

q_perm_out = q_mem*3.6e6;      %l/h
p_perm_out = 0;
c_perm_out = q_s_m/q_mem/molarMassNaCl;

s_Feed_out      = [q_feed_out, p_feed_out, c_feed_out];
s_Permeate_out  = [q_perm_out, p_perm_out, c_perm_out];

== matlab function ntw4_3_2/Fork_4_1 ==
  data: si_1 input; so_1 output; si_2 input; si_3 input; si_4 input
function so_1  = fourToOne(si_1, si_2, si_3, si_4)

q_sum = si_1(1) + si_2(1) + si_3(1) + si_4(1) ;
q_out = q_sum;

c_out  = (si_1(1)*si_1(3) + si_2(1)*si_2(3) + si_3(1)*si_3(3) + si_4(1)*si_4(3) )/q_sum;

p_out = si_1(2);

so_1 = [q_out, p_out, c_out];

== matlab function ntw4_3_2/Fork_4_3  ==
  data: si_1 input; so_1 output; si_2 input; si_3 input; si_4 input; so_2 output; so_3 output
function [so_1, so_2, so_3] = fourToThree(si_1, si_2, si_3, si_4)

q_sum = si_1(1) + si_2(1) + si_3(1) + si_4(1);
q_out = q_sum/3.0;

c_out  = (si_1(1)*si_1(3) + si_2(1)*si_2(3) + si_3(1)*si_3(3) + si_4(1)*si_4(3) )/q_sum;

p_out = si_1(2);

so_1 = [q_out, p_out, c_out];
so_2 = so_1;
so_3 = so_1;

== matlab function ntw4_3_2/RO element 5/RO Element ==
  data: s_Feed_in input; s_Permeate_out output; s_Feed_out output; memPrs input
function [s_Permeate_out, s_Feed_out] = fcn(s_Feed_in, memPrs)

% moduleParas = [d_uc, no_sht, thk_d, thk_f, thk_m, r1, r2]

% ---------------------------------fixing flow rate:
nbSheets = 20;
l_s     = 1.1;
l_l     = 0.93;

q_in    = s_Feed_in(1)/3.6*1e-6;        %m^3/s
U       = q_in/(l_s*0.711e-3*nbSheets);

dh      = 1.0673e-3;        % m
re      = U*dh*1e6;
sh      = 4.43655*re^0.48267;
D       = 1.45e-9;          % m^2/s
k_m     = sh*D/dh;        

A_m     = memPrs(1)/3.6*1e-11;  % m/s/pa
zeta    = 8.05e4;               % pa m^3/kg
molarMassNaCl   = 58.44276;     % g/mol
c_f     = s_Feed_in(3)*molarMassNaCl;       %g/l
%c_p     = s_Permeate_in(3)*molarMassNaCl;   %g/l
d_p     = s_Feed_in(2)*1e5;  % pa

a   = 0.0;
b   = 1e-4;
%fprintf('A_m = %e, dp = %e, u = %e, re = %e, k_m = %e, sh = %e\n', A_m, d_p, U, re, k_m, sh);
while abs(a-b) > 1e-10
    x   = 0.5*(a+b);
    fa  = a - A_m*(  d_p - zeta*( c_f*exp(a/k_m) )  );
    fx  = x - A_m*(  d_p - zeta*( c_f*exp(x/k_m) )  );
    %fprintf('a = %e, b = %e, x = %e, abs(a-b) = %e\n',a,b,x, abs(a-b));

    if fa*fx>0
        a   = x;
    else
        b   = x;
    end
end
jw_uc   = 0.5*(a+b);

n_s = round(l_s/(2.822e-3));
n_l = round(l_l/(2.822e-3));
area_uc = 16e-6;                %m^2
area_mod = area_uc*n_s*n_l*nbSheets;

q_mem = area_mod*jw_uc;         % m^3/s


% ---------------------------------fixing solute flux:
R_m   = memPrs(2);
q_s_m = q_mem*c_f*(1.0-R_m);    % kg/m^3, solute mass flow rate through membrane
q_s_r = (q_in*c_f - q_s_m);     % kg/m^3, solute mass flow rate retained in feed channel

% ---------------------------------fixing pressure drop:
f       = 22.91*re^-0.606;
dP      = f*U^2*1e3*l_l/(2.0*dh)*1e-5;  % bar
fprintf('f = %e\n',area_mod);

q_feed_out = (q_in-q_mem)*3.6e6 ;
p_feed_out = s_Feed_in(2) - dP;
c_feed_out = q_s_r/(q_feed_out/3.6e6)/molarMassNaCl;

q_perm_out = q_mem*3.6e6;      %l/h
p_perm_out = 0;
c_perm_out = q_s_m/q_mem/molarMassNaCl;

s_Feed_out      = [q_feed_out, p_feed_out, c_feed_out];
s_Permeate_out  = [q_perm_out, p_perm_out, c_perm_out];

== matlab function ntw4_3_2/RO element 6/RO Element ==
  data: s_Feed_in input; s_Permeate_out output; s_Feed_out output; memPrs input
function [s_Permeate_out, s_Feed_out] = fcn(s_Feed_in, memPrs)

% moduleParas = [d_uc, no_sht, thk_d, thk_f, thk_m, r1, r2]

% ---------------------------------fixing flow rate:
nbSheets = 20;
l_s     = 1.1;
l_l     = 0.93;

q_in    = s_Feed_in(1)/3.6*1e-6;        %m^3/s
U       = q_in/(l_s*0.711e-3*nbSheets);

dh      = 1.0673e-3;        % m
re      = U*dh*1e6;
sh      = 4.43655*re^0.48267;
D       = 1.45e-9;          % m^2/s
k_m     = sh*D/dh;        

A_m     = memPrs(1)/3.6*1e-11;  % m/s/pa
zeta    = 8.05e4;               % pa m^3/kg
molarMassNaCl   = 58.44276;     % g/mol
c_f     = s_Feed_in(3)*molarMassNaCl;       %g/l
%c_p     = s_Permeate_in(3)*molarMassNaCl;   %g/l
d_p     = s_Feed_in(2)*1e5;  % pa

a   = 0.0;
b   = 1e-4;
%fprintf('A_m = %e, dp = %e, u = %e, re = %e, k_m = %e, sh = %e\n', A_m, d_p, U, re, k_m, sh);
while abs(a-b) > 1e-10
    x   = 0.5*(a+b);
    fa  = a - A_m*(  d_p - zeta*( c_f*exp(a/k_m) )  );
    fx  = x - A_m*(  d_p - zeta*( c_f*exp(x/k_m) )  );
    %fprintf('a = %e, b = %e, x = %e, abs(a-b) = %e\n',a,b,x, abs(a-b));

    if fa*fx>0
        a   = x;
    else
        b   = x;
    end
end
jw_uc   = 0.5*(a+b);

n_s = round(l_s/(2.822e-3));
n_l = round(l_l/(2.822e-3));
area_uc = 16e-6;                %m^2
area_mod = area_uc*n_s*n_l*nbSheets;

q_mem = area_mod*jw_uc;         % m^3/s


% ---------------------------------fixing solute flux:
R_m   = memPrs(2);
q_s_m = q_mem*c_f*(1.0-R_m);    % kg/m^3, solute mass flow rate through membrane
q_s_r = (q_in*c_f - q_s_m);     % kg/m^3, solute mass flow rate retained in feed channel

% ---------------------------------fixing pressure drop:
f       = 22.91*re^-0.606;
dP      = f*U^2*1e3*l_l/(2.0*dh)*1e-5;  % bar
fprintf('f = %e\n',area_mod);

q_feed_out = (q_in-q_mem)*3.6e6 ;
p_feed_out = s_Feed_in(2) - dP;
c_feed_out = q_s_r/(q_feed_out/3.6e6)/molarMassNaCl;

q_perm_out = q_mem*3.6e6;      %l/h
p_perm_out = 0;
c_perm_out = q_s_m/q_mem/molarMassNaCl;

s_Feed_out      = [q_feed_out, p_feed_out, c_feed_out];
s_Permeate_out  = [q_perm_out, p_perm_out, c_perm_out];

== matlab function ntw4_3_2/RO element 7/RO Element ==
  data: s_Feed_in input; s_Permeate_out output; s_Feed_out output; memPrs input
function [s_Permeate_out, s_Feed_out] = fcn(s_Feed_in, memPrs)

% moduleParas = [d_uc, no_sht, thk_d, thk_f, thk_m, r1, r2]

% ---------------------------------fixing flow rate:
nbSheets = 20;
l_s     = 1.1;
l_l     = 0.93;

q_in    = s_Feed_in(1)/3.6*1e-6;        %m^3/s
U       = q_in/(l_s*0.711e-3*nbSheets);

dh      = 1.0673e-3;        % m
re      = U*dh*1e6;
sh      = 4.43655*re^0.48267;
D       = 1.45e-9;          % m^2/s
k_m     = sh*D/dh;        

A_m     = memPrs(1)/3.6*1e-11;  % m/s/pa
zeta    = 8.05e4;               % pa m^3/kg
molarMassNaCl   = 58.44276;     % g/mol
c_f     = s_Feed_in(3)*molarMassNaCl;       %g/l
%c_p     = s_Permeate_in(3)*molarMassNaCl;   %g/l
d_p     = s_Feed_in(2)*1e5;  % pa

a   = 0.0;
b   = 1e-4;
%fprintf('A_m = %e, dp = %e, u = %e, re = %e, k_m = %e, sh = %e\n', A_m, d_p, U, re, k_m, sh);
while abs(a-b) > 1e-10
    x   = 0.5*(a+b);
    fa  = a - A_m*(  d_p - zeta*( c_f*exp(a/k_m) )  );
    fx  = x - A_m*(  d_p - zeta*( c_f*exp(x/k_m) )  );
    %fprintf('a = %e, b = %e, x = %e, abs(a-b) = %e\n',a,b,x, abs(a-b));

    if fa*fx>0
        a   = x;
    else
        b   = x;
    end
end
jw_uc   = 0.5*(a+b);

n_s = round(l_s/(2.822e-3));
n_l = round(l_l/(2.822e-3));
area_uc = 16e-6;                %m^2
area_mod = area_uc*n_s*n_l*nbSheets;

q_mem = area_mod*jw_uc;         % m^3/s


% ---------------------------------fixing solute flux:
R_m   = memPrs(2);
q_s_m = q_mem*c_f*(1.0-R_m);    % kg/m^3, solute mass flow rate through membrane
q_s_r = (q_in*c_f - q_s_m);     % kg/m^3, solute mass flow rate retained in feed channel

% ---------------------------------fixing pressure drop:
f       = 22.91*re^-0.606;
dP      = f*U^2*1e3*l_l/(2.0*dh)*1e-5;  % bar
fprintf('f = %e\n',area_mod);

q_feed_out = (q_in-q_mem)*3.6e6 ;
p_feed_out = s_Feed_in(2) - dP;
c_feed_out = q_s_r/(q_feed_out/3.6e6)/molarMassNaCl;

q_perm_out = q_mem*3.6e6;      %l/h
p_perm_out = 0;
c_perm_out = q_s_m/q_mem/molarMassNaCl;

s_Feed_out      = [q_feed_out, p_feed_out, c_feed_out];
s_Permeate_out  = [q_perm_out, p_perm_out, c_perm_out];

== matlab function ntw4_3_2/Fork_3_2 ==
  data: si_1 input; so_1 output; si_2 input; si_3 input; so_2 output
function [so_1, so_2]  = threeToTwo(si_1, si_2, si_3)

q_sum = si_1(1) + si_2(1) + si_3(1) ;
q_out = q_sum/2.0;
c_out  = (si_1(1)*si_1(3) + si_2(1)*si_2(3) + si_3(1)*si_3(3))/q_sum;

p_out = si_1(2);

so_1 = [q_out, p_out, c_out];
so_2 = so_1;

== matlab function ntw4_3_2/Fork_3_1 ==
  data: si_1 input; so_1 output; si_2 input; si_3 input
function so_1  = threeToOne(si_1, si_2, si_3)

q_sum = si_1(1) + si_2(1) + si_3(1) ;
q_out = q_sum;
c_out  = (si_1(1)*si_1(3) + si_2(1)*si_2(3) + si_3(1)*si_3(3))/q_sum;

p_out = si_1(2);

so_1 = [q_out, p_out, c_out];

== matlab function ntw4_3_2/Fork_2_1 ==
  data: si_1 input; so_1 output; si_2 input
function so_1  = twoToOne(si_1, si_2)

q_sum = si_1(1) + si_2(1) ;
q_out = q_sum;
c_out  = (si_1(1)*si_1(3) + si_2(1)*si_2(3) )/q_sum;

p_out = si_1(2);

so_1 = [q_out, p_out, c_out];

== matlab function ntw4_3_2/Fork_2_2 ==
  data: si_1 input; so_1 output; si_2 input
function so_1  = twoToOne(si_1, si_2)

q_sum = si_1(1) + si_2(1) ;
q_out = q_sum;
c_out  = (si_1(1)*si_1(3) + si_2(1)*si_2(3) )/q_sum;

p_out = si_1(2);

so_1 = [q_out, p_out, c_out];

== matlab function ntw4_3_2/Fork_2_3 ==
  data: si_1 input; so_1 output; si_2 input
function so_1  = twoToOne(si_1, si_2)

q_sum = si_1(1) + si_2(1) ;
q_out = q_sum;
c_out  = (si_1(1)*si_1(3) + si_2(1)*si_2(3) )/q_sum;

p_out = si_1(2);

so_1 = [q_out, p_out, c_out];

== matlab function ntw4_3_2/Fork_2_4 ==
  data: si_1 input; so_1 output; si_2 input
function so_1  = twoToOne(si_1, si_2)

q_sum = si_1(1) + si_2(1) ;
q_out = q_sum;
c_out  = (si_1(1)*si_1(3) + si_2(1)*si_2(3) )/q_sum;

p_out = si_1(2);

so_1 = [q_out, p_out, c_out];
